simulink model "CessnaSim"  (R2017b)
settings: Solver=VariableStepAuto  StartTime=0.0  StopTime=simtime  RelTol=1e-4
values from neighbouring files (symbols this model uses):
  c = 4.9    [Cessna_Simulation.m]
  CDM = 0.0223    [Cessna_Simulation.m]
  CL0 = 0.307    [Cessna_Simulation.m]
  CLa = 4.41    [Cessna_Simulation.m]
  CLadot = 1.7    [Cessna_Simulation.m]
  CLDM = 0    [Cessna_Simulation.m]
  CLel = 0.43    [Cessna_Simulation.m]
  CLq = 3.9    [Cessna_Simulation.m]
  CM0R = 0.04    [Cessna_Simulation.m]
  CMadot = -7.27    [Cessna_Simulation.m]
  CMaR = -0.613    [Cessna_Simulation.m]
  CMel = -1.122    [Cessna_Simulation.m]
  CMq = -12.4    [Cessna_Simulation.m]
  eT = 0    [Cessna_Simulation.m]
  eta = 0    [Cessna_Simulation.m]
  J = 1346    [Cessna_Simulation.m]
  K = zeros(2,4)    [Cessna_Simulation.m]
  k = 0.0554    [Cessna_Simulation.m]
  m = W/g    (= 82.298136646)    [Cessna_Simulation.m]
  refState = x(1:4)    [Cessna_Simulation.m]
  rho = 2.377*10^-3    (= 0.002377)    [Cessna_Simulation.m]
  S = 174    [Cessna_Simulation.m]
  W = 2650    [Cessna_Simulation.m]
  x0 = [V0;alpha0;theta0;q0;0]    [Cessna_Simulation.m]
settings Model: Creator=stroll  LastModifiedBy=stroll
settings ModelReferenceCC: ModelReferenceMinAlgLoopOccurrences=on

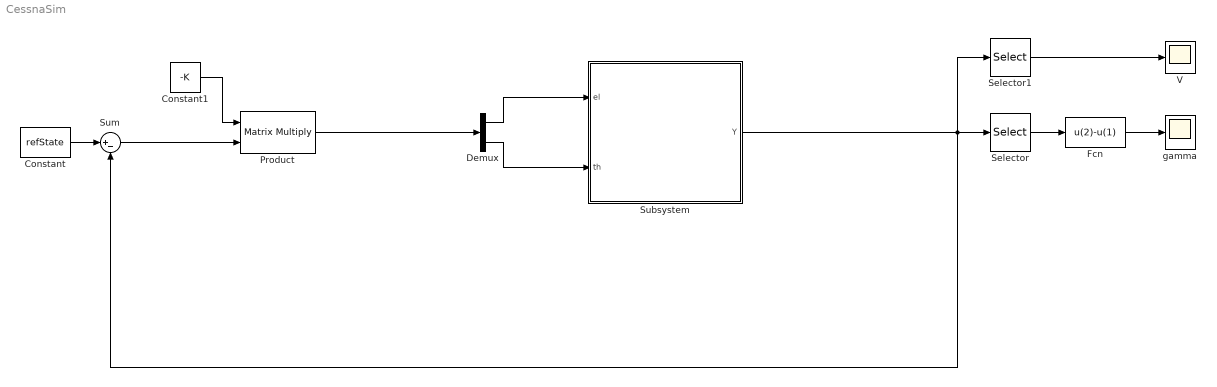
== system CessnaSim ==
  Constant : Constant  Value=refState
  Constant1 : Constant  Value=-K
  Demux : Demux  Outputs=2
  Fcn : Fcn  Expr=u(2)-u(1)
  Product : Product  Multiplication=Matrix(*)
  Selector : Selector  InputPortWidth=4  IndexOptions=Index vector (dialog)  Indices=[2 3]  OutputSizes=1
  Selector1 : Selector  InputPortWidth=4  IndexOptions=Index vector (dialog)  Indices=[1]  OutputSizes=1
  Subsystem : Subsystem
  Sum : Sum  Inputs=|+-
  V : Scope
  gamma : Scope
  wires:
  Selector1/1 -> V/1
  Demux/1 -> Subsystem/1(el)
  Demux/2 -> Subsystem/2(th)
  Constant/1 -> Sum/1
  Sum/1 -> Product/2
  Product/1 -> Demux/1
  Constant1/1 -> Product/1
  Subsystem/1(Y) -> Sum/2, Selector/1, Selector1/1
  Selector/1 -> Fcn/1
  Fcn/1 -> gamma/1

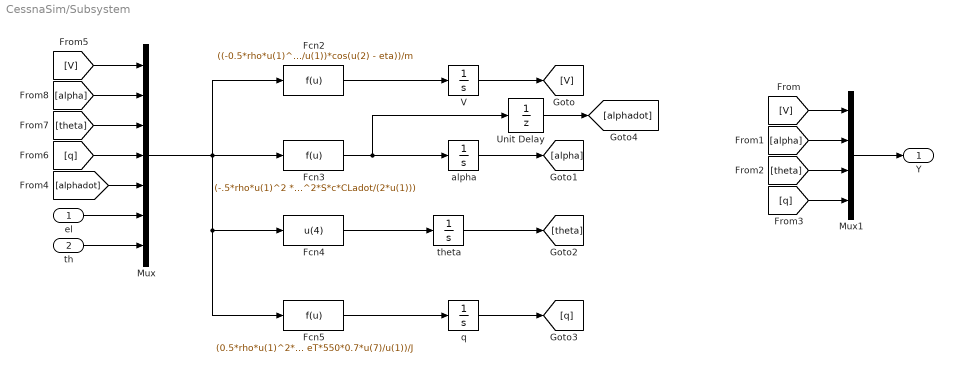
== system CessnaSim/Subsystem ==
  el : Inport
  th : Inport  Port=2
  Fcn2 : Fcn  Expr=((-0.5*rho*u(1)^2)*S*(CDM + k*(CL0 + CLa*u(2) + CLel*u(6) - CLDM)^2)-W*sin(u(3)-u(2)) + (550*u(7)*0.7/u(1))*cos(u(2) - eta))/m
  Fcn3 : Fcn  Expr=(-.5*rho*u(1)^2 *S*(CL0 + CLa*u(2) + CLel*u(6) + (c/(2*u(1)))*CLq*u(4))+W*cos(u(3)-u(2)) - (550*u(7)*0.7/u(1))*sin(u(3)-eta) + m*u(1)*u(4))/(m*u(1) + 0.5*rho*u(1)^2*S*c*CLadot/(2*u(1)))
  Fcn4 : Fcn  Expr=u(4)
  Fcn5 : Fcn  Expr=(0.5*rho*u(1)^2*S*c*(CM0R + CMaR*u(2) + CMel*u(6) + (.5*c/u(1))*(CMadot*u(5) + CMq*u(4))) + eT*550*0.7*u(7)/u(1))/J
  Mux : Mux  Inputs=7
  Mux1 : Mux
  Unit Delay : UnitDelay  SampleTime=-1
  V : Integrator  InitialCondition=x0(1)  ContinuousStateAttributes='V'
  alpha : Integrator  InitialCondition=x0(2)  ContinuousStateAttributes='alpha'
  q : Integrator  InitialCondition=x0(4)  ContinuousStateAttributes='q'
  theta : Integrator  InitialCondition=x0(3)
  Y : Outport
  wires:
  Mux1/1 -> Y/1
  [q] -> Mux1/4
  [theta] -> Mux1/3
  [theta] -> Mux/3
  Fcn3/1 -> Unit Delay/1, alpha/1
  [V] -> Mux/1
  [alphadot] -> Mux/5
  el/1 -> Mux/6
  [alpha] -> Mux/2
  Mux/1 -> Fcn2/1, Fcn4/1, Fcn5/1, Fcn3/1
  th/1 -> Mux/7
  Fcn4/1 -> theta/1
  V/1 -> [V]
  [q] -> Mux/4
  q/1 -> [q]
  Fcn5/1 -> q/1
  [V] -> Mux1/1
  alpha/1 -> [alpha]
  Fcn2/1 -> V/1
  Unit Delay/1 -> [alphadot]
  theta/1 -> [theta]
  [alpha] -> Mux1/2
